simulink model "DATA_Valid"  (R2020b)
settings: Solver=VariableStepAuto  StartTime=0.0  StopTime=10.0  RelTol=1e-3
settings Model: Creator=Nicolas  LastModifiedBy=Nicolas

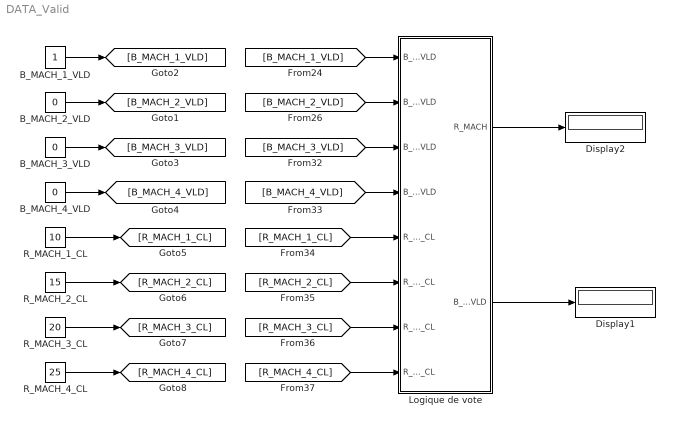
== system DATA_Valid ==
  B_MACH_1_VLD : Constant  OutDataTypeStr=single
  B_MACH_2_VLD : Constant  Value=0  OutDataTypeStr=single
  B_MACH_3_VLD : Constant  Value=0  OutDataTypeStr=single
  B_MACH_4_VLD : Constant  Value=0  OutDataTypeStr=single
  Display1 : Display
  Display2 : Display
  Logique de vote : Subsystem
  R_MACH_1_CL : Constant  Value=10  OutDataTypeStr=single
  R_MACH_2_CL : Constant  Value=15  OutDataTypeStr=single
  R_MACH_3_CL : Constant  Value=20  OutDataTypeStr=single
  R_MACH_4_CL : Constant  Value=25  OutDataTypeStr=single
  wires:
  [B_MACH_4_VLD] -> Logique de vote/4(B_MACH_4_VLD)
  B_MACH_2_VLD/1 -> [B_MACH_2_VLD]
  [B_MACH_2_VLD] -> Logique de vote/2(B_MACH_2_VLD)
  R_MACH_3_CL/1 -> [R_MACH_3_CL]
  [B_MACH_1_VLD] -> Logique de vote/1(B_MACH_1_VLD)
  [B_MACH_3_VLD] -> Logique de vote/3(B_MACH_3_VLD)
  [R_MACH_3_CL] -> Logique de vote/7(R_MACH_3_CL)
  Logique de vote/1(R_MACH) -> Display2/1
  [R_MACH_2_CL] -> Logique de vote/6(R_MACH_2_CL)
  R_MACH_2_CL/1 -> [R_MACH_2_CL]
  [R_MACH_4_CL] -> Logique de vote/8(R_MACH_4_CL)
  B_MACH_1_VLD/1 -> [B_MACH_1_VLD]
  B_MACH_4_VLD/1 -> [B_MACH_4_VLD]
  R_MACH_4_CL/1 -> [R_MACH_4_CL]
  B_MACH_3_VLD/1 -> [B_MACH_3_VLD]
  R_MACH_1_CL/1 -> [R_MACH_1_CL]
  [R_MACH_1_CL] -> Logique de vote/5(R_MACH_1_CL)
  Logique de vote/2(B_MACH_VLD) -> Display1/1

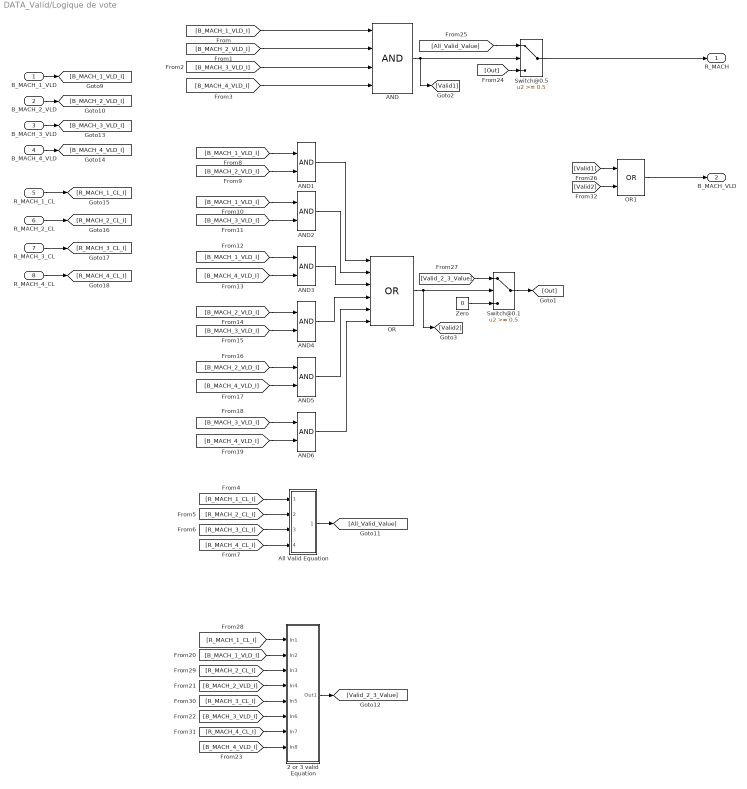
== system DATA_Valid/Logique de vote ==
  B_MACH_1_VLD : Inport
  B_MACH_2_VLD : Inport  Port=2
  B_MACH_3_VLD : Inport  Port=3
  B_MACH_4_VLD : Inport  Port=4
  R_MACH_1_CL : Inport  Port=5
  R_MACH_2_CL : Inport  Port=6
  R_MACH_3_CL : Inport  Port=7
  R_MACH_4_CL : Inport  Port=8
  2 or 3 valid Equation : Subsystem
  AND : Logic  Inputs=4  IconShape=distinctive  AllPortsSameDT=off  OutDataTypeStr=boolean
  AND{1..6} (6 alike) : Logic  IconShape=distinctive  AllPortsSameDT=off  OutDataTypeStr=boolean
  All Valid Equation : Subsystem
  OR : Logic  Operator=OR  Inputs=6  IconShape=distinctive  AllPortsSameDT=off  OutDataTypeStr=boolean
  OR1 : Logic  Operator=OR  IconShape=distinctive  AllPortsSameDT=off  OutDataTypeStr=boolean
  Switch@0.1 : Switch  Threshold=0.5
  Switch@0.5 : Switch  Threshold=0.5
  Zero : Constant  Value=0  OutDataTypeStr=single
  R_MACH : Outport
  B_MACH_VLD : Outport  Port=2
  wires:
  [B_MACH_2_VLD_I] -> AND1/2
  B_MACH_3_VLD/1 -> [B_MACH_3_VLD_I]
  [B_MACH_2_VLD_I] -> AND/2
  [B_MACH_4_VLD_I] -> AND/4
  [B_MACH_1_VLD_I] -> AND/1
  R_MACH_2_CL/1 -> [R_MACH_2_CL_I]
  [B_MACH_3_VLD_I] -> AND2/2
  R_MACH_1_CL/1 -> [R_MACH_1_CL_I]
  [R_MACH_2_CL_I] -> All Valid Equation/2(In2)
  [B_MACH_4_VLD_I] -> AND3/2
  AND2/1 -> OR/2
  [B_MACH_2_VLD_I] -> AND5/1
  [B_MACH_1_VLD_I] -> AND2/1
  [B_MACH_3_VLD_I] -> AND4/2
  [B_MACH_3_VLD_I] -> AND/3
  R_MACH_4_CL/1 -> [R_MACH_4_CL_I]
  AND4/1 -> OR/4
  B_MACH_1_VLD/1 -> [B_MACH_1_VLD_I]
  AND/1 -> [Valid1], Switch@0.5/2
  [R_MACH_4_CL_I] -> 2 or 3 valid Equation/7(In7)
  [B_MACH_3_VLD_I] -> AND6/1
  [Valid_2_3_Value] -> Switch@0.1/1
  AND5/1 -> OR/5
  OR/1 -> [Valid2], Switch@0.1/2
  [B_MACH_1_VLD_I] -> AND1/1
  [B_MACH_1_VLD_I] -> AND3/1
  [B_MACH_3_VLD_I] -> 2 or 3 valid Equation/6(In6)
  B_MACH_4_VLD/1 -> [B_MACH_4_VLD_I]
  [B_MACH_4_VLD_I] -> AND6/2
  [R_MACH_1_CL_I] -> All Valid Equation/1(In1)
  2 or 3 valid Equation/1(Out1) -> [Valid_2_3_Value]
  [R_MACH_3_CL_I] -> All Valid Equation/3(In3)
  [B_MACH_4_VLD_I] -> AND5/2
  [B_MACH_1_VLD_I] -> 2 or 3 valid Equation/2(In2)
  [R_MACH_3_CL_I] -> 2 or 3 valid Equation/5(In5)
  [R_MACH_4_CL_I] -> All Valid Equation/4(In4)
  All Valid Equation/1(Out1) -> [All_Valid_Value]
  [All_Valid_Value] -> Switch@0.5/1
  AND3/1 -> OR/3
  [R_MACH_1_CL_I] -> 2 or 3 valid Equation/1(In1)
  [B_MACH_2_VLD_I] -> 2 or 3 valid Equation/4(In4)
  [R_MACH_2_CL_I] -> 2 or 3 valid Equation/3(In3)
  AND6/1 -> OR/6
  [B_MACH_4_VLD_I] -> 2 or 3 valid Equation/8(In8)
  [B_MACH_2_VLD_I] -> AND4/1
  AND1/1 -> OR/1
  Zero/1 -> Switch@0.1/3
  R_MACH_3_CL/1 -> [R_MACH_3_CL_I]
  Switch@0.5/1 -> R_MACH/1
  B_MACH_2_VLD/1 -> [B_MACH_2_VLD_I]
  Switch@0.1/1 -> [Out]
  [Out] -> Switch@0.5/3
  [Valid1] -> OR1/1
  [Valid2] -> OR1/2
  OR1/1 -> B_MACH_VLD/1

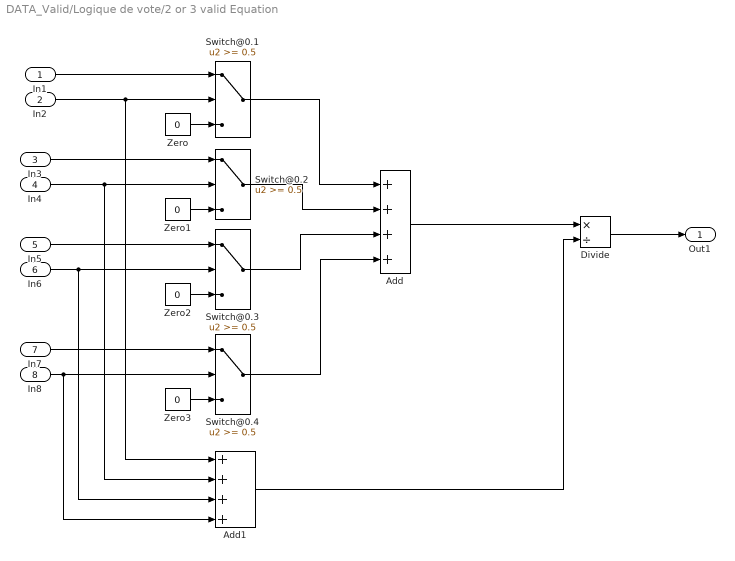
== system DATA_Valid/Logique de vote/2 or 3 valid Equation ==
  In1 : Inport
  In2 : Inport  Port=2
  In3 : Inport  Port=3
  In4 : Inport  Port=4
  In5 : Inport  Port=5
  In6 : Inport  Port=6
  In7 : Inport  Port=7
  In8 : Inport  Port=8
  Add : Sum  Inputs=++++
  Add1 : Sum  Inputs=++++
  Divide : Product  Inputs=*/
  Switch@0.{1..4} (4 alike) : Switch  Threshold=0.5
  Zero{,1..3} (4 alike) : Constant  Value=0  OutDataTypeStr=single
  Out1 : Outport
  wires:
  Add/1 -> Divide/1
  Zero3/1 -> Switch@0.4/3
  Zero/1 -> Switch@0.1/3
  Switch@0.3/1 -> Add/3
  Divide/1 -> Out1/1
  Switch@0.4/1 -> Add/4
  Zero2/1 -> Switch@0.3/3
  Zero1/1 -> Switch@0.2/3
  In1/1 -> Switch@0.1/1
  In5/1 -> Switch@0.3/1
  Switch@0.1/1 -> Add/1
  Switch@0.2/1 -> Add/2
  In3/1 -> Switch@0.2/1
  In2/1 -> Add1/1, Switch@0.1/2
  In6/1 -> Add1/3, Switch@0.3/2
  In8/1 -> Add1/4, Switch@0.4/2
  In4/1 -> Add1/2, Switch@0.2/2
  In7/1 -> Switch@0.4/1
  Add1/1 -> Divide/2

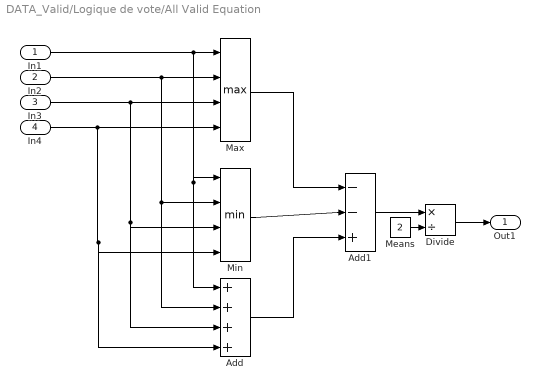
== system DATA_Valid/Logique de vote/All Valid Equation ==
  In1 : Inport
  In2 : Inport  Port=2
  In3 : Inport  Port=3
  In4 : Inport  Port=4
  Add : Sum  Inputs=++++
  Add1 : Sum  Inputs=--+
  Divide : Product  Inputs=*/
  Max : MinMax  Function=max  Inputs=4
  Means : Constant  Value=2  OutDataTypeStr=single
  Min : MinMax  Inputs=4
  Out1 : Outport
  wires:
  Add1/1 -> Divide/1
  In2/1 -> Add/2, Min/2, Max/2
  In3/1 -> Add/3, Min/3, Max/3
  Divide/1 -> Out1/1
  Means/1 -> Divide/2
  In1/1 -> Min/1, Add/1, Max/1
  In4/1 -> Add/4, Min/4, Max/4
  Max/1 -> Add1/1
  Min/1 -> Add1/2
  Add/1 -> Add1/3
